simulink model "LazoAbiertoP5"  (R2023a)
settings: Solver=ode15s  StartTime=0.0  StopTime=10  MaxStep=1e-3  RelTol=1e-3
settings Model: Creator=jesus  LastModifiedBy=jesus
settings DataIOCC: ReturnWorkspaceOutputs=off  TimeSaveName=t
settings DebuggingCC: AlgebraicLoopMsg=none  ArtificialAlgebraicLoopMsg=none  MaxConsecutiveZCsMsg=none  ModelReferenceExtraNoncontSigs=none  OperatingPointInterfaceChecksumMismatchMsg=none

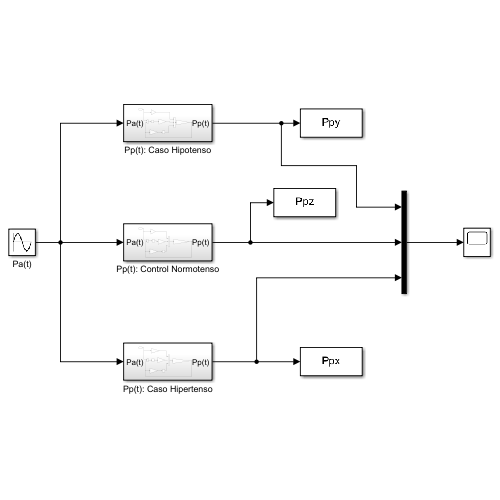
[thumbnail: Simulink's stored preview of the top-level diagram]
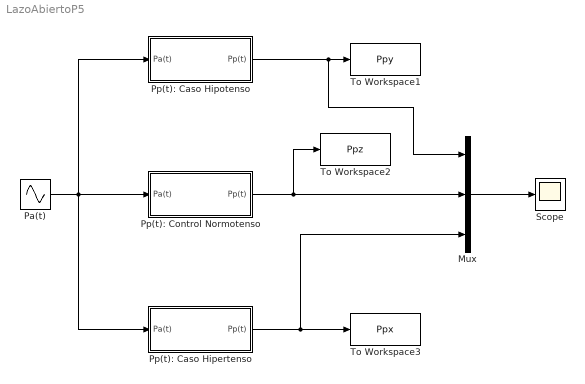
== system LazoAbiertoP5 ==
  Mux : Mux  Inputs=3
  Pa(t) : Sin  Bias=0.8  Frequency=(2*pi)*(95/60)
  Pp(t): Caso Hipertenso : Subsystem
  Pp(t): Caso Hipotenso : Subsystem
  Pp(t): Control Normotenso : Subsystem
  Scope : Scope
  To Workspace1 : ToWorkspace  VariableName=Ppy  SampleTime=-1
  To Workspace2 : ToWorkspace  VariableName=Ppz  SampleTime=-1
  To Workspace3 : ToWorkspace  VariableName=Ppx  SampleTime=-1
  wires:
  Mux/1 -> Scope/1
  Pa(t)/1 -> Pp(t): Caso Hipertenso/1(Pa(t)), Pp(t): Caso Hipotenso/1(Pa(t)), Pp(t): Control Normotenso/1(Pa(t))
  Pp(t): Caso Hipotenso/1(Pp(t)) -> To Workspace1/1, Mux/1
  Pp(t): Control Normotenso/1(Pp(t)) -> To Workspace2/1, Mux/2
  Pp(t): Caso Hipertenso/1(Pp(t)) -> To Workspace3/1, Mux/3

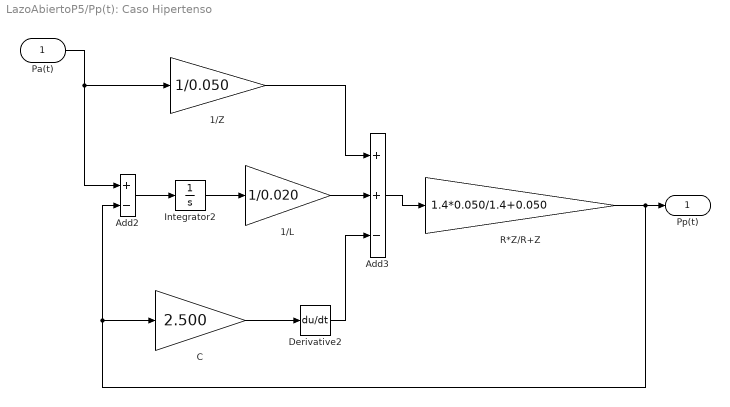
== system LazoAbiertoP5/Pp(t): Caso Hipertenso ==
  Pa(t) : Inport
  1/L : Gain  Gain=1/0.020
  1/Z : Gain  Gain=1/0.050
  Add2 : Sum  Inputs=+-
  Add3 : Sum  Inputs=++-
  C : Gain  Gain=2.500
  Derivative2 : Derivative
  Integrator2 : Integrator
  R*Z/R+Z : Gain  Gain=1.4*0.050/1.4+0.050
  Pp(t) : Outport
  wires:
  R*Z/R+Z/1 -> C/1, Add2/2, Pp(t)/1
  Derivative2/1 -> Add3/3
  C/1 -> Derivative2/1
  Pa(t)/1 -> 1/Z/1, Add2/1
  1/Z/1 -> Add3/1
  Add3/1 -> R*Z/R+Z/1
  1/L/1 -> Add3/2
  Add2/1 -> Integrator2/1
  Integrator2/1 -> 1/L/1

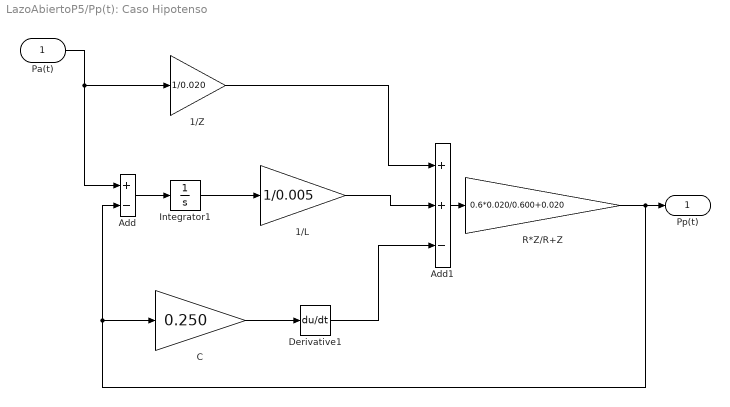
== system LazoAbiertoP5/Pp(t): Caso Hipotenso ==
  Pa(t) : Inport
  1/L : Gain  Gain=1/0.005
  1/Z : Gain  Gain=1/0.020
  Add : Sum  Inputs=+-
  Add1 : Sum  Inputs=++-
  C : Gain  Gain=0.250
  Derivative1 : Derivative
  Integrator1 : Integrator
  R*Z/R+Z : Gain  Gain=0.6*0.020/0.600+0.020
  Pp(t) : Outport
  wires:
  Derivative1/1 -> Add1/3
  R*Z/R+Z/1 -> C/1, Add/2, Pp(t)/1
  1/Z/1 -> Add1/1
  Add1/1 -> R*Z/R+Z/1
  C/1 -> Derivative1/1
  Pa(t)/1 -> Add/1, 1/Z/1
  Add/1 -> Integrator1/1
  Integrator1/1 -> 1/L/1
  1/L/1 -> Add1/2

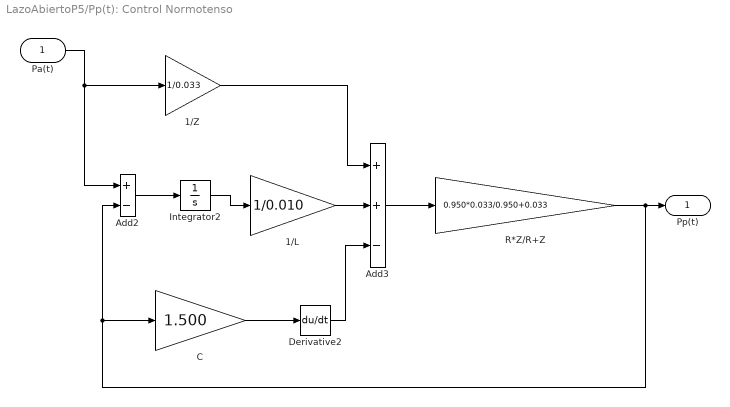
== system LazoAbiertoP5/Pp(t): Control Normotenso ==
  Pa(t) : Inport
  1/L : Gain  Gain=1/0.010
  1/Z : Gain  Gain=1/0.033
  Add2 : Sum  Inputs=+-
  Add3 : Sum  Inputs=++-
  C : Gain  Gain=1.500
  Derivative2 : Derivative
  Integrator2 : Integrator
  R*Z/R+Z : Gain  Gain=0.950*0.033/0.950+0.033
  Pp(t) : Outport
  wires:
  R*Z/R+Z/1 -> Pp(t)/1, C/1, Add2/2
  Derivative2/1 -> Add3/3
  C/1 -> Derivative2/1
  Add3/1 -> R*Z/R+Z/1
  Pa(t)/1 -> 1/Z/1, Add2/1
  1/Z/1 -> Add3/1
  1/L/1 -> Add3/2
  Add2/1 -> Integrator2/1
  Integrator2/1 -> 1/L/1
